simulink model "CF017A_GmVehPwrMod"  (R2013b)
settings: Solver=FixedStepDiscrete  SolverMode=SingleTasking  StartTime=0.0  StopTime=2  FixedStep=0.002  RelTol=1e-3
values from neighbouring files (symbols this model uses):
  ASSIKEEPMINIDX_CNT_U16 = DataDict.Constant    [CF017A_GmVehPwrMod_DataDict.m]
  BUSOFFHISPDIDX_CNT_U16 = DataDict.Constant    [CF017A_GmVehPwrMod_DataDict.m]
  CNTTOSEC_ULS_U32 = DataDict.Constant    [CF017A_GmVehPwrMod_DataDict.m]
  ENGRUNACTVIDX_CNT_U16 = DataDict.Constant    [CF017A_GmVehPwrMod_DataDict.m]
  GmVehPwrModHwTqMinKeepAssi = DataDict.Calibration    [CF017A_GmVehPwrMod_DataDict.m]
  GmVehPwrModHwTqMinKeepTmr = DataDict.Calibration    [CF017A_GmVehPwrMod_DataDict.m]
  GmVehPwrModOperRampRate = DataDict.Calibration    [CF017A_GmVehPwrMod_DataDict.m]
  GMVEHPWRMODSYSSTREQENA_CNT_LOGL = DataDict.Constant    [CF017A_GmVehPwrMod_DataDict.m]
  GMVEHPWRMODVAREFF_CNT_LOGL = DataDict.Constant    [CF017A_GmVehPwrMod_DataDict.m]
  GmVehPwrModVehSpdAssiOnMin = DataDict.Calibration    [CF017A_GmVehPwrMod_DataDict.m]
  GmVehPwrModVehSpdMinKeepAssi = DataDict.Calibration    [CF017A_GmVehPwrMod_DataDict.m]
  GPIOMCUENAIDX_CNT_U16 = DataDict.Constant    [CF017A_GmVehPwrMod_DataDict.m]
  KEEPASSIIDX_CNT_U16 = DataDict.Constant    [CF017A_GmVehPwrMod_DataDict.m]
  MSG0C9MISSIDX_CNT_U16 = DataDict.Constant    [CF017A_GmVehPwrMod_DataDict.m]
  MSG1F1MISSIDX_CNT_U16 = DataDict.Constant    [CF017A_GmVehPwrMod_DataDict.m]
  SYSPWRMODRUNIDX_CNT_U16 = DataDict.Constant    [CF017A_GmVehPwrMod_DataDict.m]
  VEHSPDSNSRVLDIDX_CNT_U16 = DataDict.Constant    [CF017A_GmVehPwrMod_DataDict.m]
libraries: simulink x2, NxtrLim x2, NxtrAbslt x1
(part 1 of 4)
settings Model: PauseTimes=2  CovMetricSettings=dcmrw  CovFilter=CF09_GMOverlayStateHandler_v002_covfilter  CovHTMLOptions=-sRT=1 -aTS=1 -bRG=1 -bTC=1 -hTR=0 -nFC=0 -scm=1 -bcm=1 -xEv=0  covSaveCumulativeToWorkspaceVar=off  CovSaveSingleToWorkspaceVar=off  CovCumulativeReport=on  Creator=SZ7VY6  LastModifiedBy=sz7vy6
settings SolverCC: AutoInsertRateTranBlk=on  InsertRTBMode=Always
settings DataIOCC: LimitDataPoints=off  SaveFormat=Structure  ReturnWorkspaceOutputs=on
settings OptimizationCC: BlockReduction=off  InlineParams=on  ZeroExternalMemoryAtStartup=off  ZeroInternalMemoryAtStartup=off  OptimizeModelRefInitCode=on  LifeSpan=1
settings DebuggingCC: SignalInfNanChecking=error  SignalRangeChecking=warning  UnderspecifiedInitializationDetection=Simplified  SolverPrmCheckMsg=error  InheritedTsInSrcMsg=error  DiscreteInheritContinuousMsg=error  SingleTaskRateTransMsg=error  TasksWithSamePriorityMsg=error  SigSpecEnsureSampleTimeMsg=error  CheckMatrixSingularityMsg=error  ParameterUnderflowMsg=error  ParameterPrecisionLossMsg=error  ParameterTunabilityLossMsg=error  FixptConstUnderflowMsg=warning  FixptConstOverflowMsg=warning  VectorMatrixConversionMsg=error  SignalLabelMismatchMsg=error  UnconnectedInputMsg=error  UnconnectedOutputMsg=error  UnconnectedLineMsg=error  SFcnCompatibilityMsg=error  UniqueDataStoreMsg=warning  BusObjectLabelMismatch=error  RootOutportRequireBusObject=error  AssertControl=DisableAll  ModelReferenceIOMsg=error  ModelReferenceVersionMismatchMessage=warning  ModelReferenceIOMismatchMessage=error  ModelReferenceCSMismatchMessage=warning  ModelReferenceDataLoggingMessage=error  StateNameClashWarn=warning  StrictBusMsg=ErrorOnBusTreatedAsVector  NonBusSignalsTreatedAsBus=error  SFUnexpectedBacktrackingDiag=error  SFInvalidInputDataAccessInChartInitDiag=error  SFNoUnconditionalDefaultTransitionDiag=error  SFTransitionOutsideNaturalParentDiag=error  SFUnconditionalTransitionShadowingDiag=error  SFUndirectedBroadcastEventsDiag=error
settings ModelReferenceCC: ModelReferenceNumInstancesAllowed=Single
settings RTWCC: SystemTargetFile=autosar.tlc  GenCodeOnly=on  TemplateMakefile=ert_default_tmf  Description=AUTOSAR  GenerateReport=on  ProcessScript=autosar_make_rtw_hook  LaunchReport=on
settings CodeAppCC: GenerateComments=off  IgnoreCustomStorageClasses=off  CustomSymbolStrType=$N$R$M  CustomSymbolStrBlkIO=$N$M  SimulinkBlockComments=off
settings STFCustomTargetCC: ParMdlRefBuildCompliant=on  CompOptLevelCompliant=on  IncludeMdlTerminateFcn=off  CombineOutputUpdateFcns=on  SuppressErrorStatus=on  ERTFirstTimeCompliant=on  ERTCustomFileBanners=on  SupportNonFinite=off  SupportComplex=off  SupportContinuousTime=off  SupportNonInlinedSFcns=off  MATLABClassNameForMDSCustomization=Simulink.SoftwareTarget.ERTCustomization  AutosarCompliant=on  GRTInterface=off  SystemTargetFile=autosar.tlc
settings ERTTargetCC: CodeReplacementLibrary=ANSI_C  ConcurrentExecutionCompliant=off  IncludeMdlTerminateFcn=off  SuppressErrorStatus=on  SupportNonFinite=off  SupportComplex=off  ModelStepFunctionPrototypeControlCompliant=off  CPPClassGenCompliant=off  AutosarCompliant=on  InlinedParameterPlacement=NonHierarchical  ERTCustomFileTemplate=example_file_process.tlc  EnableUserReplacementTypes=on

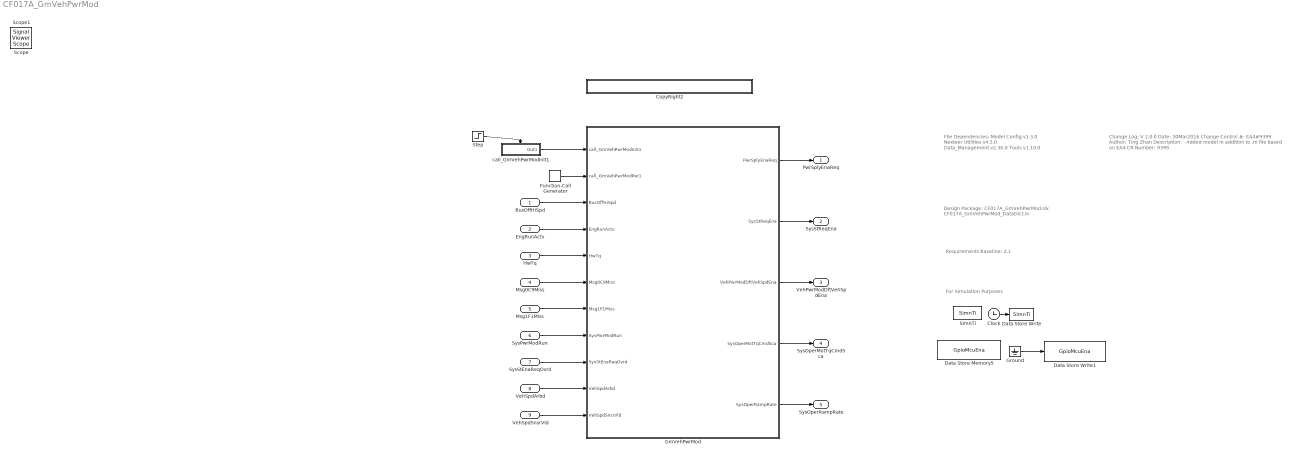
== system CF017A_GmVehPwrMod ==
  note: File Dependencies:
      |
      | Model Config v1.3.0
      | Nexteer Utilities v4.5.0
      | Data_Management v2.36.0
      | Tools v1.10.0
  note: Requirements Baseline: 2.1
  note: Change Log:
      |
      | V 2.0.0
      | Date: 30Mar2016
      | Change Control #: EA4#9399
      | Author: Ting Zhan
      | Description:
      | - Added model in addition to .m file based on EA4
      | CR Number: 9399
  note: For Simulation Purposes
  note: Design Package:
      | CF017A_GmVehPwrMod.slx
      | CF017A_GmVehPwrMod_DataDict.m
  BusOffHiSpd : Inport  RequirementInfo={} %GIDa_1b9c6812_2c02_4b85_9a2c_669458cc48bb  OutDataTypeStr=boolean
  EngRunActv : Inport  RequirementInfo={} %GIDa_f6a8d43a_8d7a_4621_b19c_bbf61fc3f1fb  Port=2  OutDataTypeStr=boolean
  HwTq : Inport  RequirementInfo={} %GIDa_8d06928a_e9dc_4bb5_bb38_60b41e7e1a37  Port=3  OutDataTypeStr=single
  Msg0C9Miss : Inport  RequirementInfo={} %GIDa_37f18a4c_7dd2_4559_8edf_851675215370  Port=4  OutDataTypeStr=boolean
  Msg1F1Miss : Inport  RequirementInfo={} %GIDa_387e051a_cae3_4bd1_96b6_4bb2f8da8f18  Port=5  OutDataTypeStr=boolean
  SysPwrModRun : Inport  RequirementInfo={} %GIDa_835686fb_41df_4b3b_981b_1312eb084a3e  Port=6  OutDataTypeStr=boolean
  SysStEnaReqOvrd : Inport  RequirementInfo={} %GIDa_951897dd_207e_4223_8bb8_db091924bf4f  Port=7  OutDataTypeStr=boolean
  VehSpdArbd : Inport  RequirementInfo={} %GIDa_a4eac490_54c7_4771_95de_17d76ce0ec27  Port=8  OutDataTypeStr=single
  VehSpdSnsrVld : Inport  RequirementInfo={} %GIDa_08a6082e_b874_4a55_b94e_1af7c22679ef  Port=9  OutDataTypeStr=boolean
  Clock : Clock
  CopyRight2 : Subsystem  Description=|  mask(Copyright Information){none=on}
      | Copyright info block.                                               
      |                                                                     
      | Place copyright information at the top of every subsystem in design.
      mask prompts: none "No parameters"
      mask help: Place copyright information at the top of every subsystem in design.
      mask Display:
      | NxtrConf = 'Nexteer Confidential';
      | 
      | sys = bdroot; %handle for the current model ("system")
      | first = get_param(sys,'Created');
      | if(isempty(first))
      |     first = datestr(now,'yyyy');
      | else
      |     first = first(end-3:end);  %year is last four digits
      | end
      | 
      | last = get_param(sys,'LastModifiedDate');
      | if isempty(last)
      |     last = datestr(now,'yyyy');
      | else
      |     last = last(end-3:end);
      | end
      | 
      | if strcmp(first,last)
      |     fprintf('%s -- Copyright %s Nexteer',NxtrConf,first)
      | else
      |     fprintf('%s -- %s%s- %s Nexteer',NxtrConf,char(169),first,last)
      | end
  Data Store Memory5 : DataStoreMemory  DataStoreName=GpioMcuEna
  Data Store Write : DataStoreWrite  DataStoreName=SimnTi
  Data Store Write1 : DataStoreWrite  DataStoreName=GpioMcuEna
  Function-Call Generator : simulink/Ports & Subsystems/Function-Call Generator  sample_time=.002  numberOfIterations=1
      settings: AttributesFormatString=%<sample_time>
  GmVehPwrMod : Subsystem
  Ground : Ground
  SimnTi : DataStoreMemory  DataStoreName=SimnTi
  Step : Step  Time=.001  Before=1  After=0  SampleTime=0
  call_GmVehPwrModInit1 : Subsystem  TreatAsAtomicUnit=on
  PwrSplyEnaReq : Outport  RequirementInfo={} %GIDa_1da87020_2114_47f8_bd6a_dcf122c70ef9
  SysStReqEna : Outport  RequirementInfo={} %GIDa_aeae8495_df44_455f_bfcb_3785565b89f3  Port=2
  VehPwrModDftVehSpdEna : Outport  RequirementInfo={} %GIDa_e60aac24_3e4f_4fa4_92d1_30c110927cae  Port=3
  SysOperMotTqCmdSca : Outport  RequirementInfo={} %GIDa_e0614fd2_7d45_427f_a7be_e9487d2cc3f6  Port=4
  SysOperRampRate : Outport  RequirementInfo={} %GIDa_71e2495b_6065_4205_97d5_a794d9935876  Port=5
  Scope : SignalViewerScope  IOType=viewer  RefreshTime=0.035000
  Scope1 : SignalViewerScope  IOType=viewer  RefreshTime=0.035000
  wires:
  Step/1 -> call_GmVehPwrModInit1/Enable
  call_GmVehPwrModInit1/1(Out1) -> GmVehPwrMod/1(call_GmVehPwrModInit1)
  Clock/1 -> Data Store Write/1
  GmVehPwrMod/1(PwrSplyEnaReq) -> PwrSplyEnaReq/1
  Function-Call Generator/1 -> GmVehPwrMod/2(call_GmVehPwrModPer1)
  GmVehPwrMod/2(SysStReqEna) -> SysStReqEna/1
  GmVehPwrMod/3(VehPwrModDftVehSpdEna) -> VehPwrModDftVehSpdEna/1
  GmVehPwrMod/4(SysOperMotTqCmdSca) -> SysOperMotTqCmdSca/1
  GmVehPwrMod/5(SysOperRampRate) -> SysOperRampRate/1
  BusOffHiSpd/1 -> GmVehPwrMod/3(BusOffHiSpd)
  EngRunActv/1 -> GmVehPwrMod/4(EngRunActv)
  HwTq/1 -> GmVehPwrMod/5(HwTq)
  Msg0C9Miss/1 -> GmVehPwrMod/6(Msg0C9Miss)
  Msg1F1Miss/1 -> GmVehPwrMod/7(Msg1F1Miss)
  SysPwrModRun/1 -> GmVehPwrMod/8(SysPwrModRun)
  SysStEnaReqOvrd/1 -> GmVehPwrMod/9(SysStEnaReqOvrd)
  VehSpdArbd/1 -> GmVehPwrMod/10(VehSpdArbd)
  VehSpdSnsrVld/1 -> GmVehPwrMod/11(VehSpdSnsrVld)
  Ground/1 -> Data Store Write1/1

== system CF017A_GmVehPwrMod/CopyRight2 ==

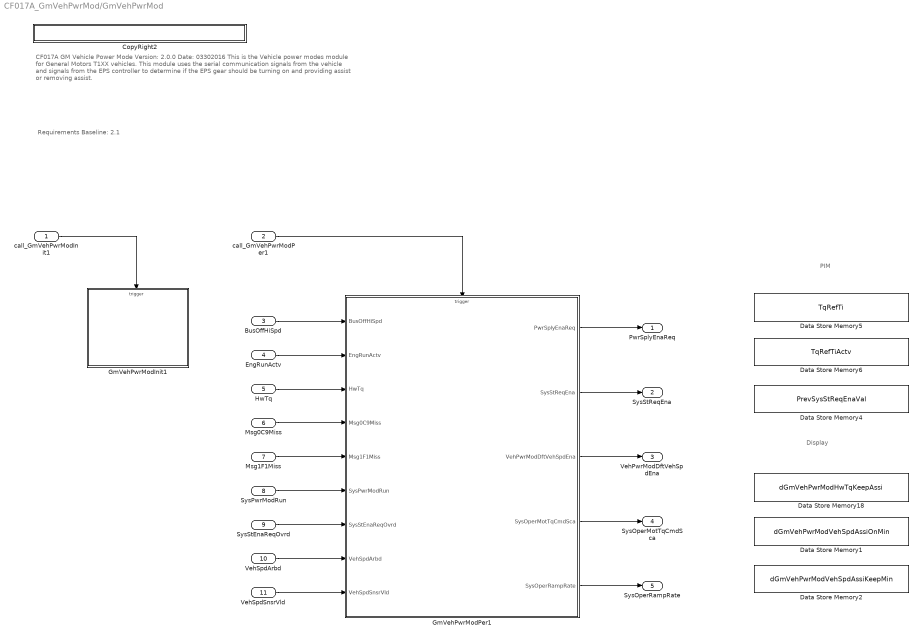
== system CF017A_GmVehPwrMod/GmVehPwrMod ==
  note: CF017A  GM Vehicle Power Mode
      | Version: 2.0.0      Date: 03302016
      |
      | This is the Vehicle power modes module for General Motors T1XX vehicles. This module uses the serial communication signals
      | from the vehicle and signals from the EPS controller to determine if the EPS gear should be turning on and providing assist or removing assist.
  note: Requirements Baseline: 2.1
  note: PIM
  note: Display
  call_GmVehPwrModInit1 : Inport  RequirementInfo={} %GIDa_bfdeb5c8_34d3_4847_8322_14533b8a1ec7
  call_GmVehPwrModPer1 : Inport  RequirementInfo={} %GIDa_f1c70cb1_f5af_488b_94e7_678758a8a022  Port=2
  BusOffHiSpd : Inport  RequirementInfo="{'linktype_rmi_doors' '0000c6e5 (/GM T1XX/SubSystem Specifications/Customer Functions/CF017A GM Vehicle Power Mode)' '#CF017A_113' 'true' 'REQ:  CF017A_113' '' } %GIDa_dae255f8_68ff_4c98_b110_bcea0aba3add"  Port=3
  EngRunActv : Inport  RequirementInfo="{'linktype_rmi_doors' '0000c6e5 (/GM T1XX/SubSystem Specifications/Customer Functions/CF017A GM Vehicle Power Mode)' '#CF017A_108' 'true' 'REQ:  CF017A_108' '' } %GIDa_f94e4f25_dea2_4ca1_8f0e_cbc76f57a275"  Port=4
  HwTq : Inport  RequirementInfo="{'linktype_rmi_doors' '0000c6e5 (/GM T1XX/SubSystem Specifications/Customer Functions/CF017A GM Vehicle Power Mode)' '#CF017A_107' 'true' 'REQ:  CF017A_107' '' } %GIDa_669e5e04_64c9_4eb9_af64_7f0439853a42"  Port=5
  Msg0C9Miss : Inport  RequirementInfo="{'linktype_rmi_doors' '0000c6e5 (/GM T1XX/SubSystem Specifications/Customer Functions/CF017A GM Vehicle Power Mode)' '#CF017A_110' 'true' 'REQ:  CF017A_110' '' } %GIDa_30a67b8a_f2de_4c81_bdbc_3e51fc1fd2c1"  Port=6
  Msg1F1Miss : Inport  RequirementInfo="{'linktype_rmi_doors' '0000c6e5 (/GM T1XX/SubSystem Specifications/Customer Functions/CF017A GM Vehicle Power Mode)' '#CF017A_112' 'true' 'REQ:  CF017A_112' '' } %GIDa_2439a840_dfd0_4d26_afae_da33f00f7dcf"  Port=7
  SysPwrModRun : Inport  RequirementInfo="{'linktype_rmi_doors' '0000c6e5 (/GM T1XX/SubSystem Specifications/Customer Functions/CF017A GM Vehicle Power Mode)' '#CF017A_42' 'true' 'REQ:  CF017A_42' '' } %GIDa_e405ee3d_6faa_40e1_bd85_7a185fe78396"  Port=8
  SysStEnaReqOvrd : Inport  RequirementInfo="{'linktype_rmi_doors' '0000c6e5 (/GM T1XX/SubSystem Specifications/Customer Functions/CF017A GM Vehicle Power Mode)' '#CF017A_129' 'true' 'REQ:  CF017A_129' '' } %GIDa_12c1b163_feda_400f_9b5a_3f16f6c62cf6"  Port=9
  VehSpdArbd : Inport  RequirementInfo="{'linktype_rmi_doors' '0000c6e5 (/GM T1XX/SubSystem Specifications/Customer Functions/CF017A GM Vehicle Power Mode)' '#CF017A_109' 'true' 'REQ:  CF017A_109' '' } %GIDa_138bcea1_08f7_4b33_bcf9_ea4f53860f30"  Port=10
  VehSpdSnsrVld : Inport  RequirementInfo="{'linktype_rmi_doors' '0000c6e5 (/GM T1XX/SubSystem Specifications/Customer Functions/CF017A GM Vehicle Power Mode)' '#CF017A_111' 'true' 'REQ:  CF017A_111' '' } %GIDa_3541169e_2345_431e_899d_04f709c184f9"  Port=11
  CopyRight2 : Subsystem  Description=|  mask(Copyright Information){none=on}
      | Copyright info block.                                               
      |                                                                     
      | Place copyright information at the top of every subsystem in design.
      mask prompts: none "No parameters"
      mask help: Place copyright information at the top of every subsystem in design.
      mask Display:
      | NxtrConf = 'Nexteer Confidential';
      | 
      | sys = bdroot; %handle for the current model ("system")
      | first = get_param(sys,'Created');
      | if(isempty(first))
      |     first = datestr(now,'yyyy');
      | else
      |     first = first(end-3:end);  %year is last four digits
      | end
      | 
      | last = get_param(sys,'LastModifiedDate');
      | if isempty(last)
      |     last = datestr(now,'yyyy');
      | else
      |     last = last(end-3:end);
      | end
      | 
      | if strcmp(first,last)
      |     fprintf('%s -- Copyright %s Nexteer',NxtrConf,first)
      | else
      |     fprintf('%s -- %s%s- %s Nexteer',NxtrConf,char(169),first,last)
      | end
  Data Store Memory1 : DataStoreMemory  DataStoreName=dGmVehPwrModVehSpdAssiOnMin  InitialValue=[]  StateMustResolveToSignalObject=on
  Data Store Memory18 : DataStoreMemory  DataStoreName=dGmVehPwrModHwTqKeepAssi  InitialValue=[]  StateMustResolveToSignalObject=on
  Data Store Memory2 : DataStoreMemory  DataStoreName=dGmVehPwrModVehSpdAssiKeepMin  InitialValue=[]  StateMustResolveToSignalObject=on
  Data Store Memory4 : DataStoreMemory  DataStoreName=PrevSysStReqEnaVal  StateMustResolveToSignalObject=on
  Data Store Memory5 : DataStoreMemory  DataStoreName=TqRefTi  StateMustResolveToSignalObject=on
  Data Store Memory6 : DataStoreMemory  DataStoreName=TqRefTiActv  StateMustResolveToSignalObject=on
  GmVehPwrModInit1 : Subsystem
  GmVehPwrModPer1 : Subsystem
  PwrSplyEnaReq : Outport  RequirementInfo="{'linktype_rmi_doors' '0000c6e5 (/GM T1XX/SubSystem Specifications/Customer Functions/CF017A GM Vehicle Power Mode)' '#CF017A_115' 'true' 'REQ:  CF017A_115' '' } %GIDa_69b1c859_cbd1_4f7d_b737_cd6829536f82"
  SysStReqEna : Outport  RequirementInfo="{'linktype_rmi_doors' '0000c6e5 (/GM T1XX/SubSystem Specifications/Customer Functions/CF017A GM Vehicle Power Mode)' '#CF017A_28' 'true' 'REQ:  CF017A_28' '' } %GIDa_7ca0a8c8_fd69_404b_8532_00ddb208e376"  Port=2
  VehPwrModDftVehSpdEna : Outport  RequirementInfo="{'linktype_rmi_doors' '0000c6e5 (/GM T1XX/SubSystem Specifications/Customer Functions/CF017A GM Vehicle Power Mode)' '#CF017A_106' 'true' 'REQ:  CF017A_106' '' } %GIDa_b6124501_08bf_46ef_9740_e78f18fd7388"  Port=3
  SysOperMotTqCmdSca : Outport  RequirementInfo="{'linktype_rmi_doors' '0000c6e5 (/GM T1XX/SubSystem Specifications/Customer Functions/CF017A GM Vehicle Power Mode)' '#CF017A_137' 'true' 'REQ:  CF017A_137' '' } %GIDa_863bbd51_b659_47ae_b395_70cee02ee7e0"  Port=4
  SysOperRampRate : Outport  RequirementInfo="{'linktype_rmi_doors' '0000c6e5 (/GM T1XX/SubSystem Specifications/Customer Functions/CF017A GM Vehicle Power Mode)' '#CF017A_138' 'true' 'REQ:  CF017A_138' '' } %GIDa_8c828841_653f_4def_a75f_5795471f1337"  Port=5
  wires:
  call_GmVehPwrModPer1/1 -> GmVehPwrModPer1/Trigger
  call_GmVehPwrModInit1/1 -> GmVehPwrModInit1/Trigger
  BusOffHiSpd/1 -> GmVehPwrModPer1/1(BusOffHiSpd)
  EngRunActv/1 -> GmVehPwrModPer1/2(EngRunActv)
  HwTq/1 -> GmVehPwrModPer1/3(HwTq)
  Msg0C9Miss/1 -> GmVehPwrModPer1/4(Msg0C9Miss)
  Msg1F1Miss/1 -> GmVehPwrModPer1/5(Msg1F1Miss)
  SysPwrModRun/1 -> GmVehPwrModPer1/6(SysPwrModRun)
  SysStEnaReqOvrd/1 -> GmVehPwrModPer1/7(SysStEnaReqOvrd)
  VehSpdArbd/1 -> GmVehPwrModPer1/8(VehSpdArbd)
  VehSpdSnsrVld/1 -> GmVehPwrModPer1/9(VehSpdSnsrVld)
  GmVehPwrModPer1/1(PwrSplyEnaReq) -> PwrSplyEnaReq/1
  GmVehPwrModPer1/2(SysStReqEna) -> SysStReqEna/1
  GmVehPwrModPer1/3(VehPwrModDftVehSpdEna) -> VehPwrModDftVehSpdEna/1
  GmVehPwrModPer1/4(SysOperMotTqCmdSca) -> SysOperMotTqCmdSca/1
  GmVehPwrModPer1/5(SysOperRampRate) -> SysOperRampRate/1

== system CF017A_GmVehPwrMod/call_GmVehPwrModInit1 ==
  Enable : EnablePort
  CopyRight2 : Subsystem  Description=|  mask(Copyright Information){none=on}
      | Copyright info block.                                               
      |                                                                     
      | Place copyright information at the top of every subsystem in design.
      mask prompts: none "No parameters"
      mask help: Place copyright information at the top of every subsystem in design.
      mask Display:
      | NxtrConf = 'Nexteer Confidential';
      | 
      | sys = bdroot; %handle for the current model ("system")
      | first = get_param(sys,'Created');
      | if(isempty(first))
      |     first = datestr(now,'yyyy');
      | else
      |     first = first(end-3:end);  %year is last four digits
      | end
      | 
      | last = get_param(sys,'LastModifiedDate');
      | if isempty(last)
      |     last = datestr(now,'yyyy');
      | else
      |     last = last(end-3:end);
      | end
      | 
      | if strcmp(first,last)
      |     fprintf('%s -- Copyright %s Nexteer',NxtrConf,first)
      | else
      |     fprintf('%s -- %s%s- %s Nexteer',NxtrConf,char(169),first,last)
      | end
  Function-Call Generator : simulink/Ports & Subsystems/Function-Call Generator  sample_time=.002  numberOfIterations=1
  Out1 : Outport
  wires:
  Function-Call Generator/1 -> Out1/1

== system CF017A_GmVehPwrMod/GmVehPwrMod/CopyRight2 ==

== system CF017A_GmVehPwrMod/GmVehPwrMod/GmVehPwrModInit1 ==
  note: Do Nothing
  function : TriggerPort  TriggerType=function-call
  CopyRight2 : Subsystem  Description=|  mask(Copyright Information){none=on}
      | Copyright info block.                                               
      |                                                                     
      | Place copyright information at the top of every subsystem in design.
      mask prompts: none "No parameters"
      mask help: Place copyright information at the top of every subsystem in design.
      mask Display:
      | NxtrConf = 'Nexteer Confidential';
      | 
      | sys = bdroot; %handle for the current model ("system")
      | first = get_param(sys,'Created');
      | if(isempty(first))
      |     first = datestr(now,'yyyy');
      | else
      |     first = first(end-3:end);  %year is last four digits
      | end
      | 
      | last = get_param(sys,'LastModifiedDate');
      | if isempty(last)
      |     last = datestr(now,'yyyy');
      | else
      |     last = last(end-3:end);
      | end
      | 
      | if strcmp(first,last)
      |     fprintf('%s -- Copyright %s Nexteer',NxtrConf,first)
      | else
      |     fprintf('%s -- %s%s- %s Nexteer',NxtrConf,char(169),first,last)
      | end

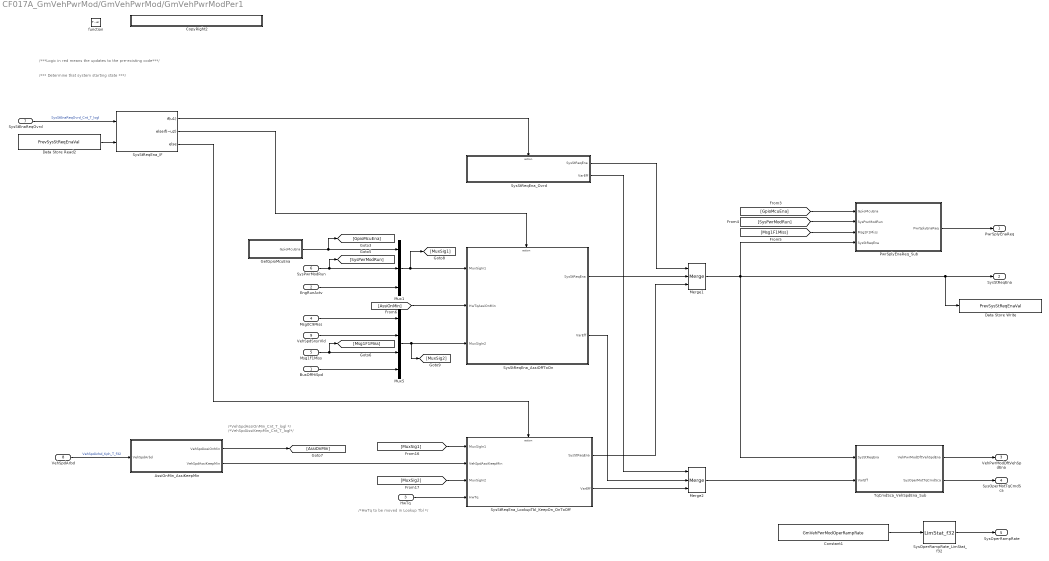
== system CF017A_GmVehPwrMod/GmVehPwrMod/GmVehPwrModPer1 ==
  note: /*** Determine that system starting state ***/
  note: /***Logic in red means the updates to the pre-existing code***/
  note: /*VehSpdAssiOnMin_Cnt_T_logl */
      | /*VehSpdAssiKeepMin_Cnt_T_logl*/
  note: /*HwTq to be moved in Lookup Tbl */
  BusOffHiSpd : Inport  RequirementInfo="{'linktype_rmi_doors' '0000c6e5 (/GM T1XX/SubSystem Specifications/Customer Functions/CF017A GM Vehicle Power Mode)' '#CF017A_130' 'true' 'REQ:  CF017A_130' '' ; 'linktype_rmi_doors' '0000c6e5 (/GM T1XX/SubSystem Specifications/Customer Functions/CF017A GM Vehicle Power Mode)' '#CF017A_132' 'true' 'REQ:  CF017A_132' '' } %GIDa_19a58a62_ea8b_42ac_976c_f323a4e5fb4e"
  EngRunActv : Inport  RequirementInfo="{'linktype_rmi_doors' '0000c6e5 (/GM T1XX/SubSystem Specifications/Customer Functions/CF017A GM Vehicle Power Mode)' '#CF017A_130' 'true' 'REQ:  CF017A_130' '' ; 'linktype_rmi_doors' '0000c6e5 (/GM T1XX/SubSystem Specifications/Customer Functions/CF017A GM Vehicle Power Mode)' '#CF017A_132' 'true' 'REQ:  CF017A_132' '' } %GIDa_c358ba99_35ee_4eda_aec4_59a7f9c2cd81"  Port=2
  HwTq : Inport  RequirementInfo="{'linktype_rmi_doors' '0000c6e5 (/GM T1XX/SubSystem Specifications/Customer Functions/CF017A GM Vehicle Power Mode)' '#CF017A_114' 'true' 'REQ:  CF017A_114' '' } %GIDa_5fab8672_ee1b_46d3_b7a0_1f2522ac3128"  Port=3
  Msg0C9Miss : Inport  RequirementInfo="{'linktype_rmi_doors' '0000c6e5 (/GM T1XX/SubSystem Specifications/Customer Functions/CF017A GM Vehicle Power Mode)' '#CF017A_130' 'true' 'REQ:  CF017A_130' '' ; 'linktype_rmi_doors' '0000c6e5 (/GM T1XX/SubSystem Specifications/Customer Functions/CF017A GM Vehicle Power Mode)' '#CF017A_132' 'true' 'REQ:  CF017A_132' '' } %GIDa_97efc4a3_badf_4f9c_a1b1_7d9397b8ff86"  Port=4
  Msg1F1Miss : Inport  RequirementInfo="{'linktype_rmi_doors' '0000c6e5 (/GM T1XX/SubSystem Specifications/Customer Functions/CF017A GM Vehicle Power Mode)' '#CF017A_130' 'true' 'REQ:  CF017A_130' '' ; 'linktype_rmi_doors' '0000c6e5 (/GM T1XX/SubSystem Specifications/Customer Functions/CF017A GM Vehicle Power Mode)' '#CF017A_132' 'true' 'REQ:  CF017A_132' '' } %GIDa_e9bf2f7a_c7b3_4dae_a4bb_9c0e9664d81c"  Port=5
  SysPwrModRun : Inport  RequirementInfo="{'linktype_rmi_doors' '0000c6e5 (/GM T1XX/SubSystem Specifications/Customer Functions/CF017A GM Vehicle Power Mode)' '#CF017A_130' 'true' 'REQ:  CF017A_130' '' ; 'linktype_rmi_doors' '0000c6e5 (/GM T1XX/SubSystem Specifications/Customer Functions/CF017A GM Vehicle Power Mode)' '#CF017A_132' 'true' 'REQ:  CF017A_132' '' } %GIDa_802be214_11fb_4c78_a748_c4be65880a91"  Port=6
  SysStEnaReqOvrd : Inport  RequirementInfo="{'linktype_rmi_doors' '0000c6e5 (/GM T1XX/SubSystem Specifications/Customer Functions/CF017A GM Vehicle Power Mode)' '#CF017A_130' 'true' 'REQ:  CF017A_130' '' ; 'linktype_rmi_doors' '0000c6e5 (/GM T1XX/SubSystem Specifications/Customer Functions/CF017A GM Vehicle Power Mode)' '#CF017A_132' 'true' 'REQ:  CF017A_132' '' ; 'linktype_rmi_doors' '0000c6e5 (/GM T1XX/SubSystem Specifications/Customer Functions/CF017A GM Vehicle Power Mode)' '#CF017A_114' 'true' 'REQ:  CF017A_114' '' ; 'linktype_rmi_doors' '0000c6e5 (/GM T1XX/SubSystem Specifications/Customer Functions/CF017A GM Vehicle Power Mode)' '#CF017A_32' 'true' 'REQ:  CF017A_32' '' } %GIDa_9436bf2b_f6f8_4f3b_879f_48b6a4552a8f"  Port=7  OutDataTypeStr=boolean
  VehSpdArbd : Inport  RequirementInfo="{'linktype_rmi_doors' '0000c6e5 (/GM T1XX/SubSystem Specifications/Customer Functions/CF017A GM Vehicle Power Mode)' '#CF017A_130' 'true' 'REQ:  CF017A_130' '' } %GIDa_751ef87e_8b73_448a_a0b2_29a8fcc2bed5"  Port=8
  VehSpdSnsrVld : Inport  RequirementInfo="{'linktype_rmi_doors' '0000c6e5 (/GM T1XX/SubSystem Specifications/Customer Functions/CF017A GM Vehicle Power Mode)' '#CF017A_130' 'true' 'REQ:  CF017A_130' '' ; 'linktype_rmi_doors' '0000c6e5 (/GM T1XX/SubSystem Specifications/Customer Functions/CF017A GM Vehicle Power Mode)' '#CF017A_132' 'true' 'REQ:  CF017A_132' '' } %GIDa_5cf324f1_224f_4a86_ab93_746adeec61c5"  Port=9
  function : TriggerPort  TriggerType=function-call
  AssiOnMin_AssiKeepMin : Subsystem
  Constant1 : Constant  RequirementInfo="{'linktype_rmi_doors' '0000c6e5 (/GM T1XX/SubSystem Specifications/Customer Functions/CF017A GM Vehicle Power Mode)' '#CF017A_142' 'true' 'REQ:  CF017A_142' '' } %GIDa_82297311_7b75_4268_b4d1_db56fef1e5c2"  Value=GmVehPwrModOperRampRate  OutDataTypeStr=single
      settings: AttributesFormatString=%<OutDataTypeStr>
  CopyRight2 : Subsystem  Description=|  mask(Copyright Information){none=on}
      | Copyright info block.                                               
      |                                                                     
      | Place copyright information at the top of every subsystem in design.
      mask prompts: none "No parameters"
      mask help: Place copyright information at the top of every subsystem in design.
      mask Display:
      | NxtrConf = 'Nexteer Confidential';
      | 
      | sys = bdroot; %handle for the current model ("system")
      | first = get_param(sys,'Created');
      | if(isempty(first))
      |     first = datestr(now,'yyyy');
      | else
      |     first = first(end-3:end);  %year is last four digits
      | end
      | 
      | last = get_param(sys,'LastModifiedDate');
      | if isempty(last)
      |     last = datestr(now,'yyyy');
      | else
      |     last = last(end-3:end);
      | end
      | 
      | if strcmp(first,last)
      |     fprintf('%s -- Copyright %s Nexteer',NxtrConf,first)
      | else
      |     fprintf('%s -- %s%s- %s Nexteer',NxtrConf,char(169),first,last)
      | end
  Data Store Read2 : DataStoreRead  RequirementInfo="{'linktype_rmi_doors' '0000c6e5 (/GM T1XX/SubSystem Specifications/Customer Functions/CF017A GM Vehicle Power Mode)' '#CF017A_130' 'true' 'REQ:  CF017A_130' '' ; 'linktype_rmi_doors' '0000c6e5 (/GM T1XX/SubSystem Specifications/Customer Functions/CF017A GM Vehicle Power Mode)' '#CF017A_132' 'true' 'REQ:  CF017A_132' '' ; 'linktype_rmi_doors' '0000c6e5 (/GM T1XX/SubSystem Specifications/Customer Functions/CF017A GM Vehicle Power Mode)' '#CF017A_114' 'true' 'REQ:  CF017A_114' '' ; 'linktype_rmi_doors' '0000c6e5 (/GM T1XX/SubSystem Specifications/Customer Functions/CF017A GM Vehicle Power Mode)' '#CF017A_32' 'true' 'REQ:  CF017A_32' '' } %GIDa_a2d83974_e587_44ec_bad0_58f9db73445f"  DataStoreName=PrevSysStReqEnaVal
  Data Store Write : DataStoreWrite  RequirementInfo="{'linktype_rmi_doors' '0000c6e5 (/GM T1XX/SubSystem Specifications/Customer Functions/CF017A GM Vehicle Power Mode)' '#CF017A_114' 'true' 'REQ:  CF017A_114' '' } %GIDa_db887a8a_e243_45b4_9f56_5e1439b1d8db"  DataStoreName=PrevSysStReqEnaVal
  GetGpioMcuEna : Subsystem
  Merge1 : Merge  RequirementInfo="{'linktype_rmi_doors' '0000c6e5 (/GM T1XX/SubSystem Specifications/Customer Functions/CF017A GM Vehicle Power Mode)' '#CF017A_32' 'true' 'REQ:  CF017A_32' '' } %GIDa_461ff05a_06f9_4a5a_b4d7_c9f5fdbb9232"  Inputs=3
  Merge2 : Merge  RequirementInfo="{'linktype_rmi_doors' '0000c6e5 (/GM T1XX/SubSystem Specifications/Customer Functions/CF017A GM Vehicle Power Mode)' '#CF017A_32' 'true' 'REQ:  CF017A_32' '' } %GIDa_3800837b_3336_44a5_a547_19f98bd0bdd6"  Inputs=3
  Mux1 : Mux  RequirementInfo="{'linktype_rmi_doors' '0000c6e5 (/GM T1XX/SubSystem Specifications/Customer Functions/CF017A GM Vehicle Power Mode)' '#CF017A_130' 'true' 'REQ:  CF017A_130' '' ; 'linktype_rmi_doors' '0000c6e5 (/GM T1XX/SubSystem Specifications/Customer Functions/CF017A GM Vehicle Power Mode)' '#CF017A_132' 'true' 'REQ:  CF017A_132' '' } %GIDa_8538414b_2453_4e81_a0f3_b9ebfcd930a3"  Inputs=3
  Mux5 : Mux  RequirementInfo="{'linktype_rmi_doors' '0000c6e5 (/GM T1XX/SubSystem Specifications/Customer Functions/CF017A GM Vehicle Power Mode)' '#CF017A_130' 'true' 'REQ:  CF017A_130' '' ; 'linktype_rmi_doors' '0000c6e5 (/GM T1XX/SubSystem Specifications/Customer Functions/CF017A GM Vehicle Power Mode)' '#CF017A_132' 'true' 'REQ:  CF017A_132' '' } %GIDa_5b13d3ae_1dd9_4bca_89a6_a8049b2fc2c5"
  PwrSplyEnaReq_Sub : Subsystem  RequirementInfo="{'linktype_rmi_doors' '0000c6e5 (/GM T1XX/SubSystem Specifications/Customer Functions/CF017A GM Vehicle Power Mode)' '#CF017A_135' 'true' 'REQ:  CF017A_135' '' } %GIDa_beac0e7d_92b8_4a67_a93b_8717eaba79b3"
  SysOperRampRate_LimStat_f32 : NxtrLim/LimStat_f32  RequirementInfo="{'linktype_rmi_doors' '0000c6e5 (/GM T1XX/SubSystem Specifications/Customer Functions/CF017A GM Vehicle Power Mode)' '#CF017A_142' 'true' 'REQ:  CF017A_142' '' } %GIDa_fd71ccfc_6824_47b9_8c9a_f8de02e9baaa"  LoLim=MINRAMPRATE_ULSPERSEC_F32  HiLim=MAXRAMPRATE_ULSPERSEC_F32
      settings: AttributesFormatString=|
      | Low Limit: %<LoLim>
      | High Limit:%<HiLim>
  SysStReqEna_AssiOffToOn : Subsystem  RequirementInfo="{'linktype_rmi_doors' '0000c6e5 (/GM T1XX/SubSystem Specifications/Customer Functions/CF017A GM Vehicle Power Mode)' '#CF017A_130' 'true' 'REQ:  CF017A_130' '' ; 'linktype_rmi_doors' '0000c6e5 (/GM T1XX/SubSystem Specifications/Customer Functions/CF017A GM Vehicle Power Mode)' '#CF017A_132' 'true' 'REQ:  CF017A_132' '' } %GIDa_3d239baa_6da6_471f_856f_eda93870d29a"  TreatAsAtomicUnit=on
  SysStReqEna_IF : If  RequirementInfo="{'linktype_rmi_doors' '0000c6e5 (/GM T1XX/SubSystem Specifications/Customer Functions/CF017A GM Vehicle Power Mode)' '#CF017A_130' 'true' 'REQ:  CF017A_130' '' ; 'linktype_rmi_doors' '0000c6e5 (/GM T1XX/SubSystem Specifications/Customer Functions/CF017A GM Vehicle Power Mode)' '#CF017A_132' 'true' 'REQ:  CF017A_132' '' ; 'linktype_rmi_doors' '0000c6e5 (/GM T1XX/SubSystem Specifications/Customer Functions/CF017A GM Vehicle Power Mode)' '#CF017A_114' 'true' 'REQ:  CF017A_114' '' ; 'linktype_rmi_doors' '0000c6e5 (/GM T1XX/SubSystem Specifications/Customer Functions/CF017A GM Vehicle Power Mode)' '#CF017A_32' 'true' 'REQ:  CF017A_32' '' } %GIDa_c13e2030_d429_45ed_a2d5_dbc0f5863a4a"  NumInputs=2  IfExpression=u1  ElseIfExpressions=~u2
      settings: AttributesFormatString=%<Priority>
  SysStReqEna_LookupTbl_KeepOn_OnToOff : Subsystem  RequirementInfo="{'linktype_rmi_doors' '0000c6e5 (/GM T1XX/SubSystem Specifications/Customer Functions/CF017A GM Vehicle Power Mode)' '#CF017A_114' 'true' 'REQ:  CF017A_114' '' } %GIDa_d4daf17d_dcfc_4103_98c7_1b0a2f52cea8"  TreatAsAtomicUnit=on
  SysStReqEna_Ovrd : Subsystem  RequirementInfo="{'linktype_rmi_doors' '0000c6e5 (/GM T1XX/SubSystem Specifications/Customer Functions/CF017A GM Vehicle Power Mode)' '#CF017A_32' 'true' 'REQ:  CF017A_32' '' } %GIDa_f8a232ed_9a21_4673_af28_86738961edba"  TreatAsAtomicUnit=on
  TqCmdSca_VehSpdEna_Sub : Subsystem
  PwrSplyEnaReq : Outport  RequirementInfo="{'linktype_rmi_doors' '0000c6e5 (/GM T1XX/SubSystem Specifications/Customer Functions/CF017A GM Vehicle Power Mode)' '#CF017A_135' 'true' 'REQ:  CF017A_135' '' } %GIDa_3e9161e8_922c_4bad_9ff1_99368e418145"
  SysStReqEna : Outport  RequirementInfo={} %GIDa_09f612c1_4377_4556_992f_978cffce312c  Port=2
  VehPwrModDftVehSpdEna : Outport  RequirementInfo={} %GIDa_73af7241_4052_4063_b947_f8759ef9a6cd  Port=3
  SysOperMotTqCmdSca : Outport  RequirementInfo={} %GIDa_0bc56f8a_5372_42b0_a0f7_ec516d4711c6  Port=4
  SysOperRampRate : Outport  RequirementInfo="{'linktype_rmi_doors' '0000c6e5 (/GM T1XX/SubSystem Specifications/Customer Functions/CF017A GM Vehicle Power Mode)' '#CF017A_142' 'true' 'REQ:  CF017A_142' '' } %GIDa_b56bfd97_0fd8_4c19_bbdb_c7407f28eb6c"  Port=5
  wires:
  SysStReqEna_IF/3 -> SysStReqEna_LookupTbl_KeepOn_OnToOff/Action
  SysStReqEna_IF/2 -> SysStReqEna_AssiOffToOn/Action
  SysPwrModRun/1 -> [SysPwrModRun], Mux1/2
  VehSpdSnsrVld/1 -> Mux5/2
  SysStReqEna_AssiOffToOn/1("SysStReqEna ") -> Merge1/2
  SysStReqEna_LookupTbl_KeepOn_OnToOff/1("SysStReqEna ") -> Merge1/3
  SysOperRampRate_LimStat_f32/1 -> SysOperRampRate/1
  Constant1/1 -> SysOperRampRate_LimStat_f32/1
  EngRunActv/1 -> Mux1/3
  [AssiOnMin] -> SysStReqEna_AssiOffToOn/2(HwTqAssiOnMin)
  BusOffHiSpd/1 -> Mux5/4
  Mux1/1 -> [MuxSig1], SysStReqEna_AssiOffToOn/1(MuxSigIn1)
  Mux5/1 -> SysStReqEna_AssiOffToOn/3(MuxSigIn2), [MuxSig2]
  Msg1F1Miss/1 -> Mux5/3, [Msg1F1Miss]
  Msg0C9Miss/1 -> Mux5/1
  [MuxSig1] -> SysStReqEna_LookupTbl_KeepOn_OnToOff/1(MuxSigIn1)
  [MuxSig2] -> SysStReqEna_LookupTbl_KeepOn_OnToOff/3(MuxSigIn2)
  [GpioMcuEna] -> PwrSplyEnaReq_Sub/1(GpioMcuEna)
  [SysPwrModRun] -> PwrSplyEnaReq_Sub/2(SysPwrModRun)
  [Msg1F1Miss] -> PwrSplyEnaReq_Sub/3(Msg1F1Miss)
  PwrSplyEnaReq_Sub/1(PwrSplyEnaReq) -> PwrSplyEnaReq/1
  SysStReqEna_LookupTbl_KeepOn_OnToOff/2(VarEff) -> Merge2/3
  TqCmdSca_VehSpdEna_Sub/1(VehPwrModDftVehSpdEna) -> VehPwrModDftVehSpdEna/1
  TqCmdSca_VehSpdEna_Sub/2(SysOperMotTqCmdSca) -> SysOperMotTqCmdSca/1
  VehSpdArbd/1 -> AssiOnMin_AssiKeepMin/1(VehSpdArbd)  "VehSpdArbd_Kph_T_f32"
  AssiOnMin_AssiKeepMin/1(VehSpdAssiOnMin) -> [AssiOnMin]
  AssiOnMin_AssiKeepMin/2(VehSpdAssiKeepMin) -> SysStReqEna_LookupTbl_KeepOn_OnToOff/2(VehSpdAssiKeepMin)
  HwTq/1 -> SysStReqEna_LookupTbl_KeepOn_OnToOff/4(HwTq)
  SysStEnaReqOvrd/1 -> SysStReqEna_IF/1  "SysStEnaReqOvrd_Cnt_T_logl"
  SysStReqEna_IF/1 -> SysStReqEna_Ovrd/Action
  SysStReqEna_Ovrd/1("SysStReqEna ") -> Merge1/1
  SysStReqEna_Ovrd/2("VarEff ") -> Merge2/1
  SysStReqEna_AssiOffToOn/2("VarEff ") -> Merge2/2
  Merge2/1 -> TqCmdSca_VehSpdEna_Sub/2(VarEff)
  Merge1/1 -> SysStReqEna/1, Data Store Write/1, TqCmdSca_VehSpdEna_Sub/1(SysStReqEna), PwrSplyEnaReq_Sub/4(SysStReqEna)
  Data Store Read2/1 -> SysStReqEna_IF/2
  GetGpioMcuEna/1(GpioMcuEna) -> [GpioMcuEna], Mux1/1

== system CF017A_GmVehPwrMod/call_GmVehPwrModInit1/CopyRight2 ==

== system CF017A_GmVehPwrMod/GmVehPwrMod/GmVehPwrModInit1/CopyRight2 ==

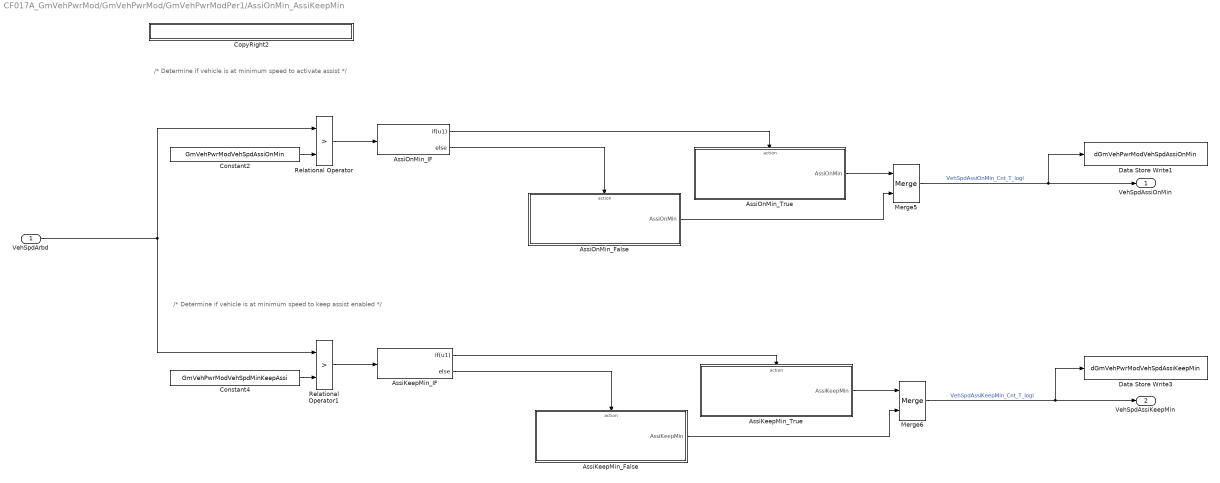
== system CF017A_GmVehPwrMod/GmVehPwrMod/GmVehPwrModPer1/AssiOnMin_AssiKeepMin ==
  note: /* Determine if vehicle is at minimum speed to activate assist */
  note: /* Determine if vehicle is at minimum speed to keep assist enabled */
  VehSpdArbd : Inport  RequirementInfo="{'linktype_rmi_doors' '0000c6e5 (/GM T1XX/SubSystem Specifications/Customer Functions/CF017A GM Vehicle Power Mode)' '#CF017A_130' 'true' 'REQ:  CF017A_130' '' ; 'linktype_rmi_doors' '0000c6e5 (/GM T1XX/SubSystem Specifications/Customer Functions/CF017A GM Vehicle Power Mode)' '#CF017A_114' 'true' 'REQ:  CF017A_114' '' } %GIDa_d690ad84_d682_4ec4_9d76_ea0929e46fbe"
  AssiKeepMin_False : Subsystem  RequirementInfo="{'linktype_rmi_doors' '0000c6e5 (/GM T1XX/SubSystem Specifications/Customer Functions/CF017A GM Vehicle Power Mode)' '#CF017A_114' 'true' 'REQ:  CF017A_114' '' } %GIDa_6bc83a35_4f13_42f4_a760_8220f50da68d"  TreatAsAtomicUnit=on
  AssiKeepMin_IF : If  RequirementInfo="{'linktype_rmi_doors' '0000c6e5 (/GM T1XX/SubSystem Specifications/Customer Functions/CF017A GM Vehicle Power Mode)' '#CF017A_114' 'true' 'REQ:  CF017A_114' '' } %GIDa_2b813240_8ed8_4791_a99c_b0339fd6fc79"  IfExpression=u1
      settings: AttributesFormatString=%<Priority>
  AssiKeepMin_True : Subsystem  RequirementInfo="{'linktype_rmi_doors' '0000c6e5 (/GM T1XX/SubSystem Specifications/Customer Functions/CF017A GM Vehicle Power Mode)' '#CF017A_114' 'true' 'REQ:  CF017A_114' '' } %GIDa_8a7ee14e_41cd_468b_a442_857eaf85b766"  TreatAsAtomicUnit=on
  AssiOnMin_False : Subsystem  RequirementInfo="{'linktype_rmi_doors' '0000c6e5 (/GM T1XX/SubSystem Specifications/Customer Functions/CF017A GM Vehicle Power Mode)' '#CF017A_130' 'true' 'REQ:  CF017A_130' '' } %GIDa_021087e3_b1cc_416e_93df_1e1190829e6c"  TreatAsAtomicUnit=on
  AssiOnMin_IF : If  RequirementInfo="{'linktype_rmi_doors' '0000c6e5 (/GM T1XX/SubSystem Specifications/Customer Functions/CF017A GM Vehicle Power Mode)' '#CF017A_130' 'true' 'REQ:  CF017A_130' '' } %GIDa_4912aaac_3459_4007_9a78_f8edcb52d835"  IfExpression=u1
      settings: AttributesFormatString=%<Priority>
  AssiOnMin_True : Subsystem  RequirementInfo="{'linktype_rmi_doors' '0000c6e5 (/GM T1XX/SubSystem Specifications/Customer Functions/CF017A GM Vehicle Power Mode)' '#CF017A_130' 'true' 'REQ:  CF017A_130' '' } %GIDa_9d615f88_a2f9_47c9_979d_68cc32c8b087"  TreatAsAtomicUnit=on
  Constant2 : Constant  RequirementInfo="{'linktype_rmi_doors' '0000c6e5 (/GM T1XX/SubSystem Specifications/Customer Functions/CF017A GM Vehicle Power Mode)' '#CF017A_130' 'true' 'REQ:  CF017A_130' '' } %GIDa_ee923566_9f25_45de_843d_923b4f1abef3"  Value=GmVehPwrModVehSpdAssiOnMin  OutDataTypeStr=single
      settings: AttributesFormatString=%<OutDataTypeStr>
  Constant4 : Constant  RequirementInfo="{'linktype_rmi_doors' '0000c6e5 (/GM T1XX/SubSystem Specifications/Customer Functions/CF017A GM Vehicle Power Mode)' '#CF017A_114' 'true' 'REQ:  CF017A_114' '' } %GIDa_8faa65f4_fa6c_433b_a9d6_5b13fe40a4e7"  Value=GmVehPwrModVehSpdMinKeepAssi  OutDataTypeStr=single
      settings: AttributesFormatString=%<OutDataTypeStr>
  CopyRight2 : Subsystem  Description=|  mask(Copyright Information){none=on}
      | Copyright info block.                                               
      |                                                                     
      | Place copyright information at the top of every subsystem in design.
      mask prompts: none "No parameters"
      mask help: Place copyright information at the top of every subsystem in design.
      mask Display:
      | NxtrConf = 'Nexteer Confidential';
      | 
      | sys = bdroot; %handle for the current model ("system")
      | first = get_param(sys,'Created');
      | if(isempty(first))
      |     first = datestr(now,'yyyy');
      | else
      |     first = first(end-3:end);  %year is last four digits
      | end
      | 
      | last = get_param(sys,'LastModifiedDate');
      | if isempty(last)
      |     last = datestr(now,'yyyy');
      | else
      |     last = last(end-3:end);
      | end
      | 
      | if strcmp(first,last)
      |     fprintf('%s -- Copyright %s Nexteer',NxtrConf,first)
      | else
      |     fprintf('%s -- %s%s- %s Nexteer',NxtrConf,char(169),first,last)
      | end
  Data Store Write1 : DataStoreWrite  DataStoreName=dGmVehPwrModVehSpdAssiOnMin
  Data Store Write3 : DataStoreWrite  DataStoreName=dGmVehPwrModVehSpdAssiKeepMin
  Merge5 : Merge  RequirementInfo="{'linktype_rmi_doors' '0000c6e5 (/GM T1XX/SubSystem Specifications/Customer Functions/CF017A GM Vehicle Power Mode)' '#CF017A_130' 'true' 'REQ:  CF017A_130' '' } %GIDa_72413f3f_927a_4cd1_800f_fec500ff6798"
  Merge6 : Merge  RequirementInfo="{'linktype_rmi_doors' '0000c6e5 (/GM T1XX/SubSystem Specifications/Customer Functions/CF017A GM Vehicle Power Mode)' '#CF017A_114' 'true' 'REQ:  CF017A_114' '' } %GIDa_a37e385a_47e1_4dca_b975_e5ad134a975e"
  Relational Operator : RelationalOperator  RequirementInfo="{'linktype_rmi_doors' '0000c6e5 (/GM T1XX/SubSystem Specifications/Customer Functions/CF017A GM Vehicle Power Mode)' '#CF017A_130' 'true' 'REQ:  CF017A_130' '' } %GIDa_0972d201_c821_4ae0_a31e_2620590e8ab6"  Operator=>  OutDataTypeStr=boolean
  Relational Operator1 : RelationalOperator  RequirementInfo="{'linktype_rmi_doors' '0000c6e5 (/GM T1XX/SubSystem Specifications/Customer Functions/CF017A GM Vehicle Power Mode)' '#CF017A_114' 'true' 'REQ:  CF017A_114' '' } %GIDa_6bdd092a_ee8f_4c78_b89c_1f219545e8fa"  Operator=>  OutDataTypeStr=boolean
  VehSpdAssiOnMin : Outport  RequirementInfo="{'linktype_rmi_doors' '0000c6e5 (/GM T1XX/SubSystem Specifications/Customer Functions/CF017A GM Vehicle Power Mode)' '#CF017A_130' 'true' 'REQ:  CF017A_130' '' } %GIDa_f5e1363e_a317_4f2f_9b9d_5cc61d7223fd"
  VehSpdAssiKeepMin : Outport  RequirementInfo="{'linktype_rmi_doors' '0000c6e5 (/GM T1XX/SubSystem Specifications/Customer Functions/CF017A GM Vehicle Power Mode)' '#CF017A_114' 'true' 'REQ:  CF017A_114' '' } %GIDa_543184b4_848f_4d1b_b144_000c3e503d6f"  Port=2
  wires:
  Constant2/1 -> Relational Operator/2
  VehSpdArbd/1 -> Relational Operator/1, Relational Operator1/1
  Relational Operator/1 -> AssiOnMin_IF/1
  Constant4/1 -> Relational Operator1/2
  Relational Operator1/1 -> AssiKeepMin_IF/1
  AssiOnMin_IF/1 -> AssiOnMin_True/Action
  AssiOnMin_IF/2 -> AssiOnMin_False/Action
  AssiOnMin_True/1("AssiOnMin ") -> Merge5/1
  Merge5/1 -> VehSpdAssiOnMin/1, Data Store Write1/1  "VehSpdAssiOnMin_Cnt_T_logl"
  AssiOnMin_False/1("AssiOnMin ") -> Merge5/2
  AssiKeepMin_IF/1 -> AssiKeepMin_True/Action
  AssiKeepMin_IF/2 -> AssiKeepMin_False/Action
  AssiKeepMin_True/1("AssiKeepMin ") -> Merge6/1
  AssiKeepMin_False/1("AssiKeepMin ") -> Merge6/2
  Merge6/1 -> Data Store Write3/1, VehSpdAssiKeepMin/1  "VehSpdAssiKeepMin_Cnt_T_logl"

== system CF017A_GmVehPwrMod/GmVehPwrMod/GmVehPwrModPer1/CopyRight2 ==

== system CF017A_GmVehPwrMod/GmVehPwrMod/GmVehPwrModPer1/GetGpioMcuEna ==
  CopyRight2 : Subsystem  Description=|  mask(Copyright Information){none=on}
      | Copyright info block.                                               
      |                                                                     
      | Place copyright information at the top of every subsystem in design.
      mask prompts: none "No parameters"
      mask help: Place copyright information at the top of every subsystem in design.
      mask Display:
      | NxtrConf = 'Nexteer Confidential';
      | 
      | sys = bdroot; %handle for the current model ("system")
      | first = get_param(sys,'Created');
      | if(isempty(first))
      |     first = datestr(now,'yyyy');
      | else
      |     first = first(end-3:end);  %year is last four digits
      | end
      | 
      | last = get_param(sys,'LastModifiedDate');
      | if isempty(last)
      |     last = datestr(now,'yyyy');
      | else
      |     last = last(end-3:end);
      | end
      | 
      | if strcmp(first,last)
      |     fprintf('%s -- Copyright %s Nexteer',NxtrConf,first)
      | else
      |     fprintf('%s -- %s%s- %s Nexteer',NxtrConf,char(169),first,last)
      | end
  Data Store Read1 : DataStoreRead  DataStoreName=GpioMcuEna
  GpioMcuEna : Outport
  wires:
  Data Store Read1/1 -> GpioMcuEna/1

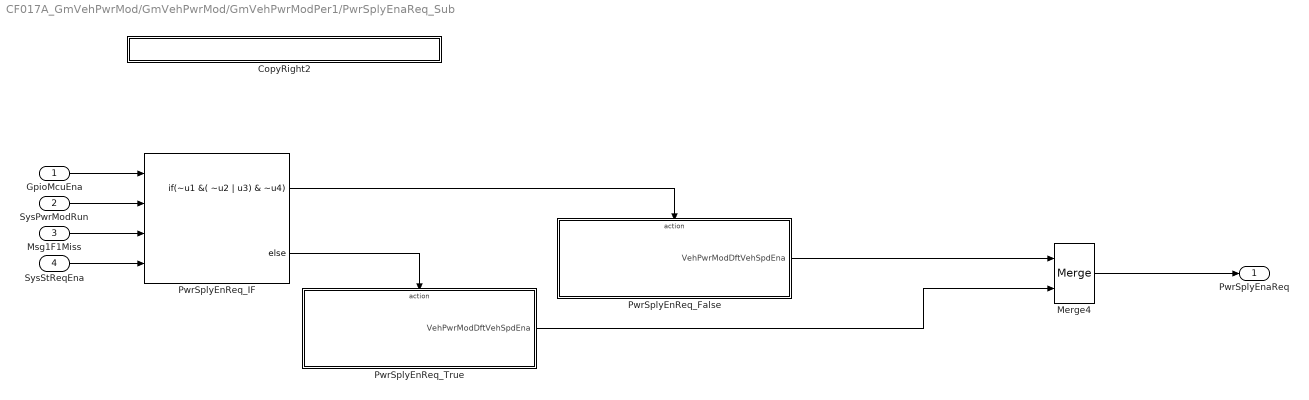
== system CF017A_GmVehPwrMod/GmVehPwrMod/GmVehPwrModPer1/PwrSplyEnaReq_Sub ==
  GpioMcuEna : Inport  RequirementInfo="{'linktype_rmi_doors' '0000c6e5 (/GM T1XX/SubSystem Specifications/Customer Functions/CF017A GM Vehicle Power Mode)' '#CF017A_135' 'true' 'REQ:  CF017A_135' '' } %GIDa_ae3d7106_f554_40b7_bbf4_4b0327f91963"
  SysPwrModRun : Inport  RequirementInfo="{'linktype_rmi_doors' '0000c6e5 (/GM T1XX/SubSystem Specifications/Customer Functions/CF017A GM Vehicle Power Mode)' '#CF017A_135' 'true' 'REQ:  CF017A_135' '' } %GIDa_2a3906ec_ad6c_477d_97a6_cc9b5304db36"  Port=2
  Msg1F1Miss : Inport  RequirementInfo="{'linktype_rmi_doors' '0000c6e5 (/GM T1XX/SubSystem Specifications/Customer Functions/CF017A GM Vehicle Power Mode)' '#CF017A_135' 'true' 'REQ:  CF017A_135' '' } %GIDa_b1a60ccf_1f1f_4a58_b445_55885429371f"  Port=3
  SysStReqEna : Inport  RequirementInfo="{'linktype_rmi_doors' '0000c6e5 (/GM T1XX/SubSystem Specifications/Customer Functions/CF017A GM Vehicle Power Mode)' '#CF017A_135' 'true' 'REQ:  CF017A_135' '' } %GIDa_91697371_f3cc_4584_b7e9_124963939fbe"  Port=4
  CopyRight2 : Subsystem  Description=|  mask(Copyright Information){none=on}
      | Copyright info block.                                               
      |                                                                     
      | Place copyright information at the top of every subsystem in design.
      mask prompts: none "No parameters"
      mask help: Place copyright information at the top of every subsystem in design.
      mask Display:
      | NxtrConf = 'Nexteer Confidential';
      | 
      | sys = bdroot; %handle for the current model ("system")
      | first = get_param(sys,'Created');
      | if(isempty(first))
      |     first = datestr(now,'yyyy');
      | else
      |     first = first(end-3:end);  %year is last four digits
      | end
      | 
      | last = get_param(sys,'LastModifiedDate');
      | if isempty(last)
      |     last = datestr(now,'yyyy');
      | else
      |     last = last(end-3:end);
      | end
      | 
      | if strcmp(first,last)
      |     fprintf('%s -- Copyright %s Nexteer',NxtrConf,first)
      | else
      |     fprintf('%s -- %s%s- %s Nexteer',NxtrConf,char(169),first,last)
      | end
  Merge4 : Merge  RequirementInfo="{'linktype_rmi_doors' '0000c6e5 (/GM T1XX/SubSystem Specifications/Customer Functions/CF017A GM Vehicle Power Mode)' '#CF017A_135' 'true' 'REQ:  CF017A_135' '' } %GIDa_09906b9e_70d7_41ac_b979_829c769c8287"
  PwrSplyEnReq_False : Subsystem  RequirementInfo="{'linktype_rmi_doors' '0000c6e5 (/GM T1XX/SubSystem Specifications/Customer Functions/CF017A GM Vehicle Power Mode)' '#CF017A_135' 'true' 'REQ:  CF017A_135' '' } %GIDa_38d841ce_dbe3_4a44_8c88_3da2d060f349"  TreatAsAtomicUnit=on
  PwrSplyEnReq_IF : If  RequirementInfo="{'linktype_rmi_doors' '0000c6e5 (/GM T1XX/SubSystem Specifications/Customer Functions/CF017A GM Vehicle Power Mode)' '#CF017A_135' 'true' 'REQ:  CF017A_135' '' } %GIDa_ab4105e2_aa37_4164_a751_01f04b6c92a5"  NumInputs=4  IfExpression=~u1 &( ~u2 | u3) & ~u4
      settings: AttributesFormatString=IF: %<IfExpression>
  PwrSplyEnReq_True : Subsystem  RequirementInfo="{'linktype_rmi_doors' '0000c6e5 (/GM T1XX/SubSystem Specifications/Customer Functions/CF017A GM Vehicle Power Mode)' '#CF017A_135' 'true' 'REQ:  CF017A_135' '' } %GIDa_d9f15c9e_6978_4581_a300_e63d17a89bef"  TreatAsAtomicUnit=on
  PwrSplyEnaReq : Outport  RequirementInfo="{'linktype_rmi_doors' '0000c6e5 (/GM T1XX/SubSystem Specifications/Customer Functions/CF017A GM Vehicle Power Mode)' '#CF017A_135' 'true' 'REQ:  CF017A_135' '' } %GIDa_26435abe_7af3_4d5c_8d99_5f9400f14cc8"
  wires:
  Merge4/1 -> PwrSplyEnaReq/1
  GpioMcuEna/1 -> PwrSplyEnReq_IF/1
  SysPwrModRun/1 -> PwrSplyEnReq_IF/2
  Msg1F1Miss/1 -> PwrSplyEnReq_IF/3
  PwrSplyEnReq_IF/1 -> PwrSplyEnReq_False/Action
  PwrSplyEnReq_IF/2 -> PwrSplyEnReq_True/Action
  PwrSplyEnReq_False/1("VehPwrModDftVehSpdEna ") -> Merge4/1
  PwrSplyEnReq_True/1("VehPwrModDftVehSpdEna ") -> Merge4/2
  SysStReqEna/1 -> PwrSplyEnReq_IF/4
